simulink model "skipperLQR"  (R2024b)
settings: Solver=VariableStepAuto  StartTime=0.0  StopTime=100  RelTol=1e-3
InitFcn:
  | % Get state-space and gain matrices.
  | [A, B, C, D, K] = lqrMatrices(1, 10, 1/4, 1, 1, 1, 10, NaN)
values from neighbouring files (symbols this model uses):
  A = [0 0 0 1 0 0 0 0 0 0 0 0 ... (first row only)    [EOMStateSpace.m]    (also in EOMStateSpaceTest.m = [0 1 0 0 0 0 0 0 0 0 0 0; EOMStateSpaceWithConstants.m = [0 0 0 0 0            0          1 0 0 0 0 0 0; eomStateSpace.m = zeros(12, 12); lqrMatrices.m = zeros(12, 12))
  B = [0 0 0 0 0 ... (first row only)    [EOMStateSpace.m]    (also in EOMStateSpaceTest.m = [0 0 0 0; EOMStateSpaceWithConstants.m = [0   0    0     0; eomStateSpace.m = zeros(12, 5); lqrMatrices.m = zeros(12, 4))
  C = diag(ones(1, 12))    [EOMStateSpace.m]    (also in EOMStateSpaceTest.m = [1 0 0 0 0 0 0 0 0 0 0 0; EOMStateSpaceWithConstants.m = diag(ones(1, 13)); eomStateSpace.m; lqrMatrices.m)
  D = zeros(size(B))    [EOMStateSpace.m]    (also in EOMStateSpaceTest.m = [0 0 0 0; EOMStateSpaceWithConstants.m; eomStateSpace.m; lqrMatrices.m)
  K = lqr(sys, Q, R)    [eomStateSpace.m]    (also in lqrMatrices.m)
settings Model: Creator=nehir  LastModifiedBy=nehir

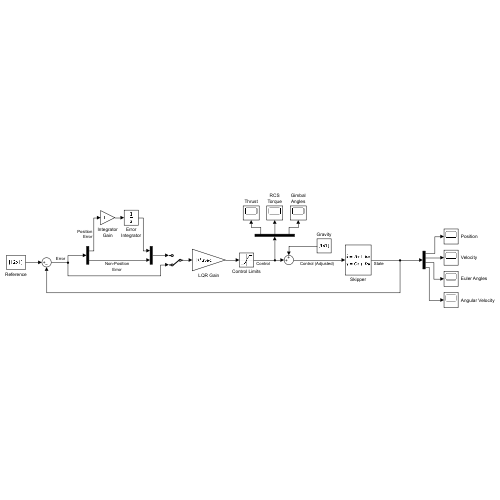
[thumbnail: Simulink's stored preview of the top-level diagram]
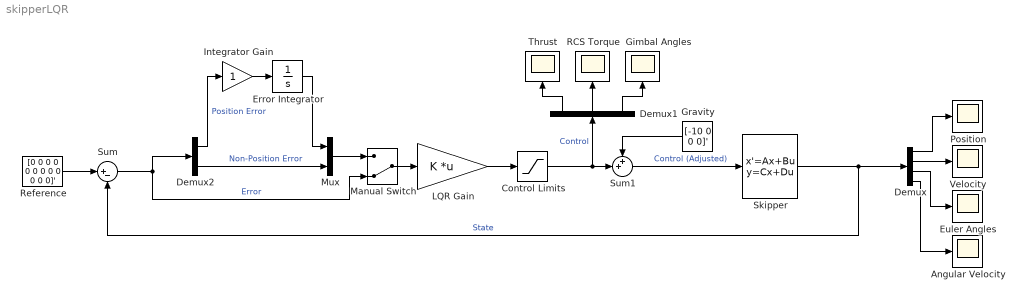
== system skipperLQR ==
  Angular Velocity : Scope
  Control Limits : Saturate  UpperLimit=[15 1 pi/18 pi/18]'  LowerLimit=[0 -1 -pi/18 -pi/18]'
  Demux : Demux  Outputs=[3 3 3 3]
  Demux1 : Demux  Outputs=[1 1 2]
  Demux2 : Demux  Outputs=[1 11]
  Error Integrator : Integrator
  Euler Angles : Scope
  Gimbal Angles : Scope
  Gravity : Constant  Value=[-10 0 0 0]'
  Integrator Gain : Gain
  LQR Gain : Gain  Gain=K  Multiplication=Matrix(K*u) (u vector)  OutDataTypeStr=double
  Manual Switch : ManualSwitch  CurrentSetting=0
  Mux : Mux  Inputs=2
  Position : Scope
  RCS Torque : Scope
  Reference : Constant  Value=[0 0 0 0 0 0 0 0 0 0 0 0]'
  Skipper : StateSpace  A=A  B=B  C=C  D=D  InitialCondition=[0 0 0 0 0 0 0 0 0 0 0 0]'
  Sum : Sum  Inputs=|+-
  Sum1 : Sum  Inputs=++|
  Thrust : Scope
  "Velocity " : Scope
  wires:
  Sum1/1 -> Skipper/1  "Control (Adjusted)"
  Skipper/1 -> Sum/2, Demux/1  "State"
  Sum/1 -> Manual Switch/2, Demux2/1  "Error"
  Demux1/2 -> RCS Torque/1
  Demux1/1 -> Thrust/1
  Demux1/3 -> Gimbal Angles/1
  Demux/1 -> Position/1
  Demux/2 -> "Velocity "/1
  Demux/3 -> Euler Angles/1
  Demux/4 -> Angular Velocity/1
  Reference/1 -> Sum/1
  Gravity/1 -> Sum1/1
  Control Limits/1 -> Sum1/2, Demux1/1  "Control"
  LQR Gain/1 -> Control Limits/1
  Error Integrator/1 -> Mux/1
  Demux2/1 -> Integrator Gain/1  "Position Error"
  Integrator Gain/1 -> Error Integrator/1
  Demux2/2 -> Mux/2  "Non-Position Error"
  Mux/1 -> Manual Switch/1
  Manual Switch/1 -> LQR Gain/1
